simulink model "ME322_Exercise_2_Simulink"  (R2024b)
settings: Solver=VariableStepAuto  StartTime=0.0  StopTime=10.0  RelTol=1e-6
undefined symbols (not defined in the file): A, A_r, B, b_s, b_t, C, D, k_s, k_t, lambda_r, m_c, m_u, xdot_c
settings Model: Creator=caidenbonney  LastModifiedBy=Caide

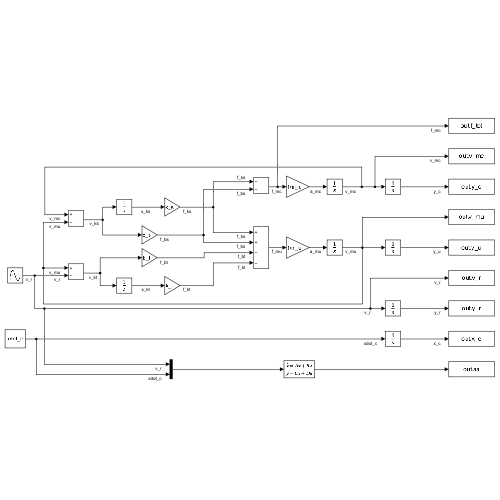
[thumbnail: Simulink's stored preview of the top-level diagram]
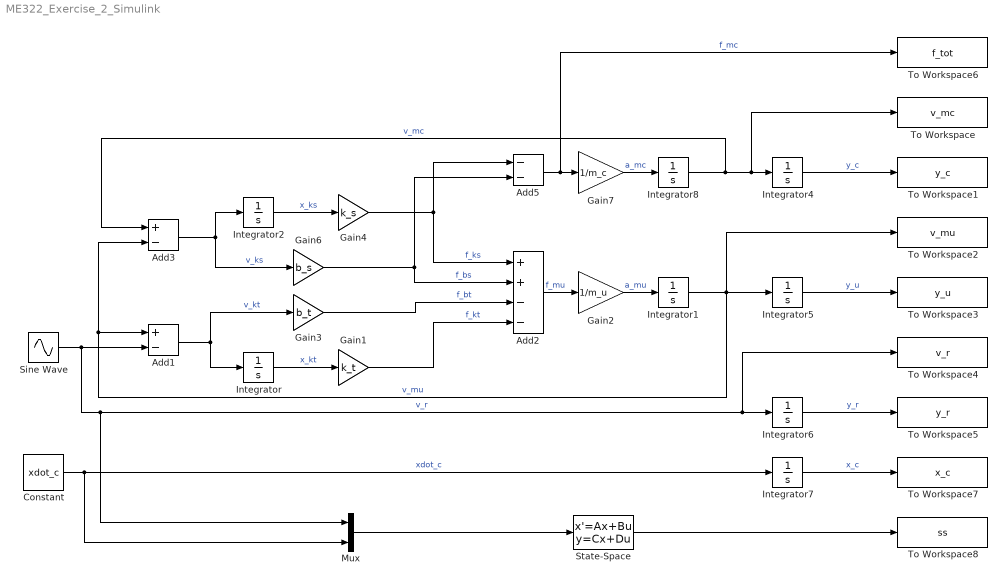
== system ME322_Exercise_2_Simulink ==
  Add1 : Sum  Inputs=+-
  Add2 : Sum  Inputs=++--
  Add3 : Sum  Inputs=+-
  Add5 : Sum  Inputs=--
  Constant : Constant  Value=xdot_c
  Gain1 : Gain  Gain=k_t
  Gain2 : Gain  Gain=1/m_u
  Gain3 : Gain  Gain=b_t
  Gain4 : Gain  Gain=k_s
  Gain6 : Gain  Gain=b_s
  Gain7 : Gain  Gain=1/m_c
  Integrator{,1..2,4..8} (8 alike) : Integrator
  Mux : Mux  Inputs=2
  Sine Wave : Sin  Amplitude=(2*pi()*A_r*xdot_c)/lambda_r  Frequency=(2*pi()*xdot_c)/lambda_r  Phase=pi()/2  SampleTime=0
  State-Space : StateSpace  A=A  B=B  C=C  D=D  InitialCondition=0
  To Workspace : ToWorkspace  VariableName=v_mc  SampleTime=-1
  To Workspace1 : ToWorkspace  VariableName=y_c  SampleTime=-1
  To Workspace2 : ToWorkspace  VariableName=v_mu  SampleTime=-1
  To Workspace3 : ToWorkspace  VariableName=y_u  SampleTime=-1
  To Workspace4 : ToWorkspace  VariableName=v_r  SampleTime=-1
  To Workspace5 : ToWorkspace  VariableName=y_r  SampleTime=-1
  To Workspace6 : ToWorkspace  VariableName=f_tot  SampleTime=-1
  To Workspace7 : ToWorkspace  VariableName=x_c  SampleTime=-1
  To Workspace8 : ToWorkspace  VariableName=ss  SampleTime=-1
  wires:
  Integrator/1 -> Gain1/1  "x_kt"
  Gain3/1 -> Add2/3  "f_bt"
  Integrator1/1 -> To Workspace2/1, Integrator5/1, Add1/1, Add3/2  "v_mu"
  Integrator8/1 -> Integrator4/1, To Workspace/1, Add3/1  "v_mc"
  Gain6/1 -> Add5/2, Add2/2  "f_bs"
  Integrator2/1 -> Gain4/1  "x_ks"
  Add1/1 -> Gain3/1, Integrator/1  "v_kt"
  Gain1/1 -> Add2/4  "f_kt"
  Add2/1 -> Gain2/1  "f_mu"
  Add3/1 -> Gain6/1, Integrator2/1  "v_ks"
  Gain4/1 -> Add2/1, Add5/1  "f_ks"
  Add5/1 -> Gain7/1, To Workspace6/1  "f_mc"
  Sine Wave/1 -> To Workspace4/1, Integrator6/1, Mux/1, Add1/2  "v_r"
  Integrator5/1 -> To Workspace3/1  "y_u"
  Integrator4/1 -> To Workspace1/1  "y_c"
  Integrator6/1 -> To Workspace5/1  "y_r"
  Constant/1 -> Integrator7/1, Mux/2  "xdot_c"
  Integrator7/1 -> To Workspace7/1  "x_c"
  Gain2/1 -> Integrator1/1  "a_mu"
  Gain7/1 -> Integrator8/1  "a_mc"
  Mux/1 -> State-Space/1
  State-Space/1 -> To Workspace8/1
